simulink model "IP_nonLinearSys_LQG"  (R2015a)
settings: Solver=ode5  StartTime=0.0  StopTime=20  FixedStep=0.01  RelTol=1e-3
settings Model: Creator=Fares  LastModifiedBy=Fares

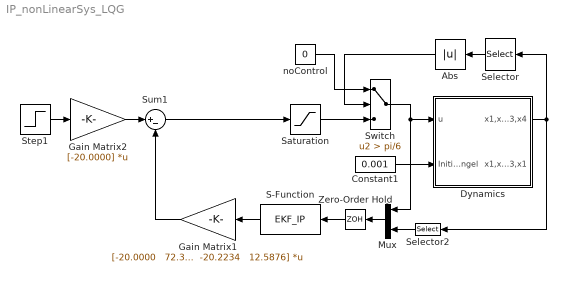
== system IP_nonLinearSys_LQG ==
  Abs : Abs
  Constant1 : Constant  Value=0.001
  Dynamics : Subsystem  mask{mc=1.12, mpw=0.095, mps=0.025, M=9.4, fp=0.000107443, J=0.013935418, l=0.033245968, g=9.81}
      mask prompts: mc "Cart mass [kg]"; mpw "Pendulum weight mass [kg]"; mps "Pendulum stick mass [kg]"; M "Maximum control [N]"; fp "Pendulum friction [kg*m2/s]"; J "Moment of inertia [kg*m2]"; l "Distance: axis of rotation-mass center [m]"; g "Gravetational acceleration [m/s2]"
      mask init:
      | mp = mpw + mps;
      | a = l^2 + J/(mc + mp);
      | mi = (mc + mp)*l;
      mask Display: plot([0],[-2.5],[5],[4.5],[0 5],[0 0],[0 5],[0.1 0.1],[0 2],[1 1],[2.5 5],[1 1],[2 2.5 2.5 2 2],[1.25 1.25 0.75 0.75 1.25],[2.25 1.5],[1 -2.5]);
  Gain Matrix1 : Gain  Gain="[-20.0000   72.3354  -20.2234   12.5876]"  Multiplication=Matrix(K*u) (u vector)
  Gain Matrix2 : Gain  Gain=[-20.0000]  Multiplication=Matrix(K*u) (u vector)
  Mux : Mux  Inputs=2
  S-Function : S-Function  FunctionName=EKF_IP  Parameters=0.01
  Saturation : Saturate  UpperLimit=2.5  LowerLimit=-2.5
  Selector : Selector  InputPortWidth=4  Indices=[2]
  Selector2 : Selector  InputPortWidth=4  Indices=[1]
  Step1 : Step  Time=10  After=0.2  SampleTime=0
  Sum1 : Sum  Inputs=|+-
  Switch : Switch  Criteria=u2 > Threshold  Threshold=pi/6
  Zero-Order Hold : ZeroOrderHold  SampleTime=0.01
  noControl : Constant  Value=0
  wires:
  Abs/1 -> Switch/2
  noControl/1 -> Switch/1
  Saturation/1 -> Switch/3
  Selector/1 -> Abs/1
  Constant1/1 -> Dynamics/2(Initial_Angel)
  S-Function/1 -> Gain Matrix1/1
  Dynamics/1(x1,x2,x3,x4) -> Selector2/1, Selector/1
  Step1/1 -> Gain Matrix2/1
  Sum1/1 -> Saturation/1
  Selector2/1 -> Mux/2
  Mux/1 -> Zero-Order Hold/1
  Zero-Order Hold/1 -> S-Function/1
  Switch/1 -> Dynamics/1(u), Mux/1
  Gain Matrix1/1 -> Sum1/2
  Gain Matrix2/1 -> Sum1/1

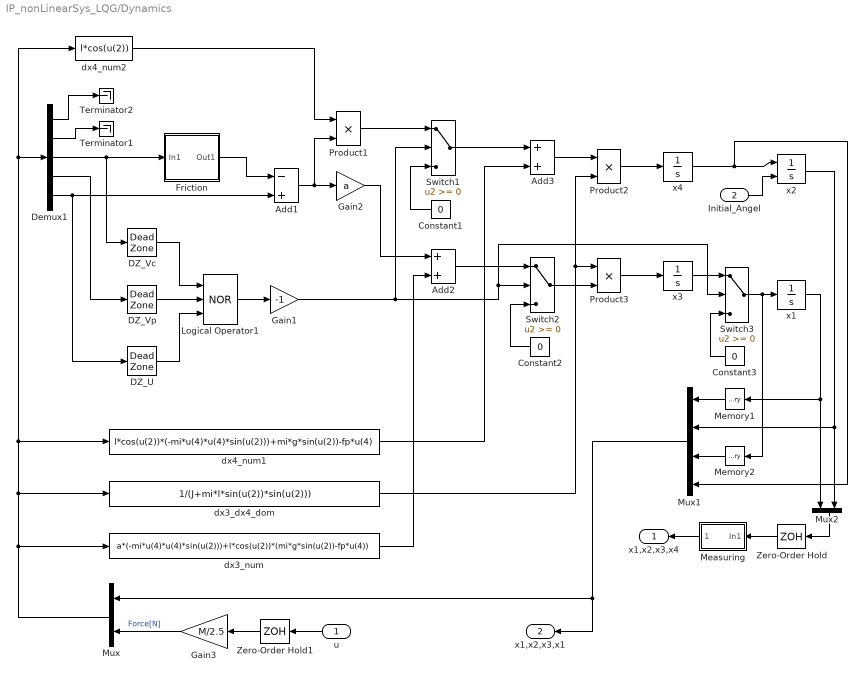
== system IP_nonLinearSys_LQG/Dynamics ==
  u : Inport
  Initial_Angel : Inport  Port=2
  " DZ_Vp" : DeadZone  LowerValue=-3.37476  UpperValue=3.37476  SaturateOnIntegerOverflow=on
  Add1 : Sum  Inputs=-+
  Add2 : Sum
  Add3 : Sum
  Constant1 : Constant  Value=0
  Constant2 : Constant  Value=0
  Constant3 : Constant  Value=0
  DZ_U : DeadZone  LowerValue=-1.37918  UpperValue=1.37918  SaturateOnIntegerOverflow=on
  DZ_Vc : DeadZone  LowerValue=-0.00793711  UpperValue=0.00793711  SaturateOnIntegerOverflow=on
  Demux1 : Demux  Outputs=5
  Friction : Subsystem  mask{FS=2.53165, FC=2.28133, DZcv=0.00793711, Xc=0.9, Yc=2.3}
      mask prompts: FS "Static friction [N]"; FC "Coulombic friction [N]"; DZcv "Minimum cart velocity [rad/s]"; Xc "Cart velocity - beginning of the linear dependence zone [m/s]"; Yc "Friction value for Xc point [N]"
      mask init:
      | small = DZcv;
      mask Display: plot([-4 4],[0 0],[-3.8 -2.4 -1.8 -1.2 -0.6 -0.2 0 0.2 0.6 1.2 1.8 2.4 3.8],[-1.4 -1 -1.1 -1.3 -1.6 -2 0 2 1.6 1.3 1.1 1 1.4]);
  Gain1 : Gain  Gain=-1
  Gain2 : Gain  Gain=a
  Gain3 : Gain  Gain=M/2.5
  Logical Operator1 : Logic  Operator=NOR  Inputs=3  AllPortsSameDT=off  OutDataTypeStr=boolean
  Measuring : Subsystem
  Memory1 : Memory
  Memory2 : Memory
  Mux : Mux  Inputs=2
  Mux1 : Mux
  Mux2 : Mux  Inputs=2
  Product1 : Product
  Product2 : Product
  Product3 : Product
  Switch1 : Switch
  Switch2 : Switch
  Switch3 : Switch
  Terminator1 : Terminator
  Terminator2 : Terminator
  Zero-Order Hold : ZeroOrderHold  SampleTime=0.01
  Zero-Order Hold1 : ZeroOrderHold  SampleTime=0.01
  dx3_dx4_dom : Fcn  Expr=1/(J+mi*l*sin(u(2))*sin(u(2)))
  dx3_num : Fcn  Expr=a*(-mi*u(4)*u(4)*sin(u(2)))+l*cos(u(2))*(mi*g*sin(u(2))-fp*u(4))
  dx4_num1 : Fcn  Expr=l*cos(u(2))*(-mi*u(4)*u(4)*sin(u(2)))+mi*g*sin(u(2))-fp*u(4)
  dx4_num2 : Fcn  Expr=l*cos(u(2))
  x1 : Integrator
  x2 : Integrator  InitialConditionSource=external  InitialCondition=pi/2
  x3 : Integrator
  x4 : Integrator
  x1,x2,x3,x4 : Outport
  x1,x2,x3,x1 : Outport  Port=2
  wires:
  DZ_U/1 -> Logical Operator1/3
  DZ_Vc/1 -> Logical Operator1/1
  Product1/1 -> Switch1/1
  Gain2/1 -> Add2/1
  Constant1/1 -> Switch1/3
  Switch2/1 -> Product3/2
  Product3/1 -> x3/1
  Logical Operator1/1 -> Gain1/1
  Constant3/1 -> Switch3/3
  Add3/1 -> Product2/1
  Demux1/1 -> Terminator2/1
  Mux/1 -> dx3_dx4_dom/1, dx4_num2/1, Demux1/1, dx4_num1/1, dx3_num/1
  dx4_num1/1 -> Add3/2
  x3/1 -> Switch3/1
  Switch3/1 -> Memory2/1, x1/1
  Add1/1 -> Gain2/1, Product1/2
  Add2/1 -> Switch2/1
  dx4_num2/1 -> Product1/1
  Demux1/3 -> Friction/1(In1), DZ_Vc/1
  Demux1/2 -> Terminator1/1
  Demux1/4 -> " DZ_Vp"/1
  Demux1/5 -> Add1/2, DZ_U/1
  " DZ_Vp"/1 -> Logical Operator1/2
  Switch1/1 -> Add3/1
  dx3_num/1 -> Add2/2
  Constant2/1 -> Switch2/3
  dx3_dx4_dom/1 -> Product2/2, Product3/1
  Product2/1 -> x4/1
  x4/1 -> x2/1, Mux1/4
  Memory2/1 -> Mux1/3
  Memory1/1 -> Mux1/1
  Mux1/1 -> x1,x2,x3,x1/1, Mux/1
  u/1 -> Zero-Order Hold1/1
  Friction/1(Out1) -> Add1/1
  Initial_Angel/1 -> x2/2
  Gain1/1 -> Switch1/2, Switch3/2, Switch2/2
  x2/1 -> Mux2/2, Mux1/2
  x1/1 -> Mux2/1, Memory1/1
  Measuring/1(Out1) -> x1,x2,x3,x4/1
  Mux2/1 -> Zero-Order Hold/1
  Zero-Order Hold/1 -> Measuring/1(In1)
  Zero-Order Hold1/1 -> Gain3/1
  Gain3/1 -> Mux/2  "Force[N]"

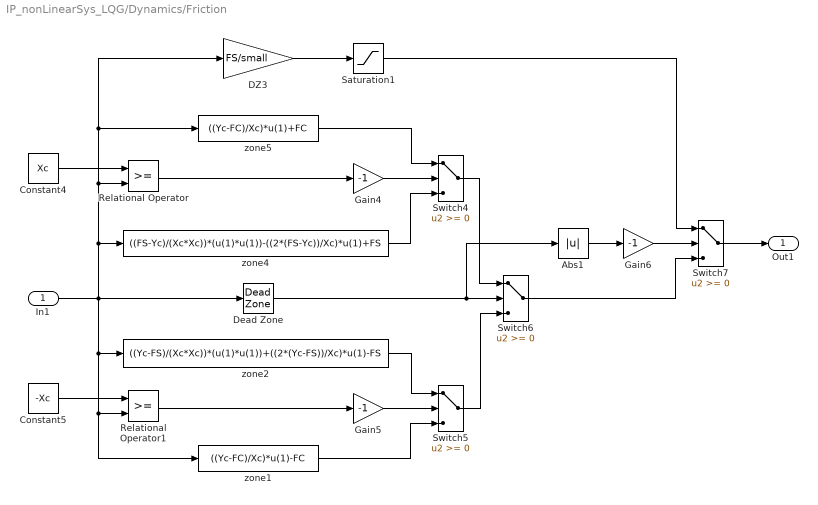
== system IP_nonLinearSys_LQG/Dynamics/Friction ==
  In1 : Inport
  Abs1 : Abs
  Constant4 : Constant  Value=Xc
  Constant5 : Constant  Value=-Xc
  DZ3 : Gain  Gain=FS/small
  Dead Zone : DeadZone  LowerValue=-DZcv  UpperValue=DZcv  SaturateOnIntegerOverflow=on
  Gain4 : Gain  Gain=-1
  Gain5 : Gain  Gain=-1
  Gain6 : Gain  Gain=-1
  Relational Operator : RelationalOperator  OutDataTypeStr=boolean
  Relational Operator1 : RelationalOperator  OutDataTypeStr=boolean
  Saturation1 : Saturate  UpperLimit=FS  LowerLimit=-FS
  Switch{4..7} (4 alike) : Switch
  zone1 : Fcn  Expr=((Yc-FC)/Xc)*u(1)-FC
  zone2 : Fcn  Expr=((Yc-FS)/(Xc*Xc))*(u(1)*u(1))+((2*(Yc-FS))/Xc)*u(1)-FS
  zone4 : Fcn  Expr=((FS-Yc)/(Xc*Xc))*(u(1)*u(1))-((2*(FS-Yc))/Xc)*u(1)+FS
  zone5 : Fcn  Expr=((Yc-FC)/Xc)*u(1)+FC
  Out1 : Outport
  wires:
  Gain4/1 -> Switch4/2
  Dead Zone/1 -> Abs1/1, Switch6/2
  Gain5/1 -> Switch5/2
  Relational Operator/1 -> Gain4/1
  Constant5/1 -> Relational Operator1/1
  Relational Operator1/1 -> Gain5/1
  Abs1/1 -> Gain6/1
  DZ3/1 -> Saturation1/1
  Switch6/1 -> Switch7/3
  Switch4/1 -> Switch6/1
  zone2/1 -> Switch5/1
  Gain6/1 -> Switch7/2
  zone4/1 -> Switch4/3
  Switch7/1 -> Out1/1
  In1/1 -> zone1/1, Relational Operator1/2, zone2/1, DZ3/1, zone5/1, Relational Operator/2, zone4/1, Dead Zone/1
  Saturation1/1 -> Switch7/1
  zone5/1 -> Switch4/1
  Constant4/1 -> Relational Operator/1
  zone1/1 -> Switch5/3
  Switch5/1 -> Switch6/3

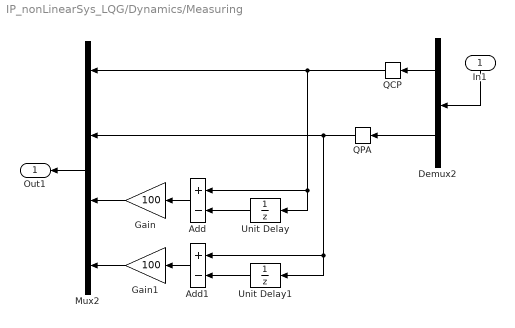
== system IP_nonLinearSys_LQG/Dynamics/Measuring ==
  In1 : Inport
  Add : Sum  Inputs=+-
  Add1 : Sum  Inputs=+-
  Demux2 : Demux  Outputs=2
  Gain : Gain  Gain=100
  Gain1 : Gain  Gain=100
  Mux2 : Mux
  QCP : Quantizer  QuantizationInterval=0.156/2048
  QPA : Quantizer  QuantizationInterval=(2*pi)/2048
  Unit Delay : UnitDelay  SampleTime=-1
  Unit Delay1 : UnitDelay  SampleTime=-1
  Out1 : Outport
  wires:
  Demux2/1 -> QCP/1
  Mux2/1 -> Out1/1
  In1/1 -> Demux2/1
  QPA/1 -> Unit Delay1/1, Add1/1, Mux2/2
  QCP/1 -> Unit Delay/1, Add/1, Mux2/1
  Demux2/2 -> QPA/1
  Unit Delay1/1 -> Add1/2
  Unit Delay/1 -> Add/2
  Add1/1 -> Gain1/1
  Add/1 -> Gain/1
  Gain1/1 -> Mux2/4
  Gain/1 -> Mux2/3
